simulink model "Attitude_Control"  (R2018b)
settings: Solver=VariableStepAuto  StartTime=0.0  StopTime=500.0  RelTol=1e-3  EnableMultiTasking=on
undefined symbols (not defined in the file): qd
libraries: Satellite_Dynamics x1, PD_Controller_Lib x1
settings Model: Creator=devantormey  LastModifiedBy=devantormey
settings OptimizationCC: LifeSpan=inf
settings DebuggingCC: SFUnexpectedBacktrackingDiag=warning  SFNoUnconditionalDefaultTransitionDiag=warning
settings SFSimCC: SimUseLocalCustomCode=off
settings RTWCC: RTWUseLocalCustomCode=off
settings CodeAppCC: StateflowObjectComments=on
settings GRTTargetCC: TargetLangStandard=C89/C90 (ANSI)  GeneratePreprocessorConditionals=Disable all
settings ConfigComp: CovMetricSettings=dw  CovHtmlReporting=on  CovSaveCumulativeToWorkspaceVar=on  CovSaveSingleToWorkspaceVar=on  CovExternalEMLEnable=off

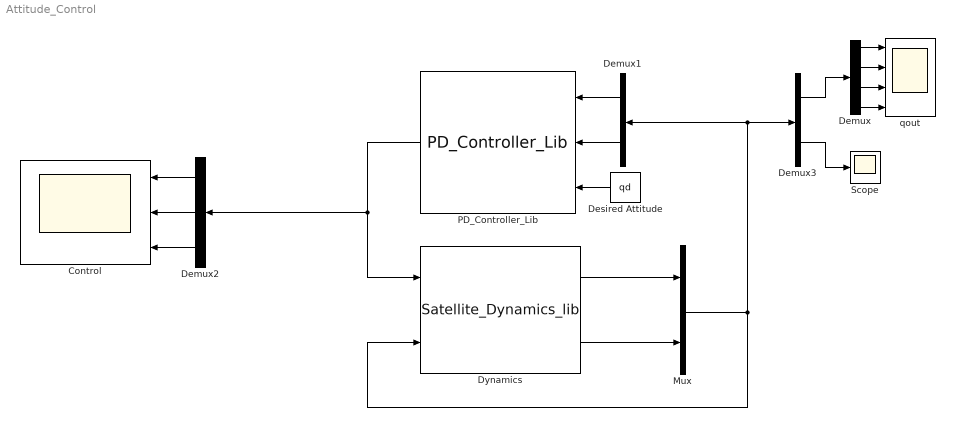
== system Attitude_Control ==
  Control : Scope  NumInputPorts=3
  Demux : Demux
  Demux1 : Demux  Outputs=[4 3]
  Demux2 : Demux  Outputs=3
  Demux3 : Demux  Outputs=[4 3]
  Desired Attitude : Constant  Value=qd
  "Dynamics " : Satellite_Dynamics/Satellite_Dynamics_lib  SystemSampleTime=-1
      link override Constant: Value=J
  Mux : Mux  Inputs=[4 3]
  PD_Controller_Lib : PD_Controller_Lib/PD_Controller_Lib  SystemSampleTime=-1
  Scope : Scope
  qout : Scope  NumInputPorts=4
  wires:
  Demux/1 -> qout/1
  Demux/2 -> qout/2
  Demux/3 -> qout/3
  Demux/4 -> qout/4
  PD_Controller_Lib/1 -> Demux2/1, "Dynamics "/1
  Demux2/2 -> Control/2
  Demux2/1 -> Control/1
  Demux2/3 -> Control/3
  Desired Attitude/1 -> PD_Controller_Lib/3
  Mux/1 -> Demux3/1, Demux1/1, "Dynamics "/2
  "Dynamics "/2 -> Mux/2
  "Dynamics "/1 -> Mux/1
  Demux1/1 -> PD_Controller_Lib/1
  Demux1/2 -> PD_Controller_Lib/2
  Demux3/1 -> Demux/1
  Demux3/2 -> Scope/1
